simulink model "MIMO_model"  (R2018b)
settings: Solver=FixedStepAuto  StartTime=0.0  StopTime=Tmod  FixedStep=0.01  RelTol=1e-3
values from neighbouring files (symbols this model uses):
  denominator11 = FormDenominator(T1_11, T2_11, T3_11, flag11)    [Graph.m]    (also in KombRegNominalOU.m = FormDenominator(T1, T2, T3, flag); KombRobAdReg.m; KombRobReg.m; MIMONominalReg.m)
  denominator12 = FormDenominator(T1_12, T2_12, T3_12, flag12)    [Graph.m]    (also in KombRegNominalOU.m = FormDenominator(T1, T2, T3, flag); KombRobAdReg.m; KombRobReg.m; MIMONominalReg.m)
  denominator21 = FormDenominator(T1_21, T2_21, T3_21, flag21)    [Graph.m]    (also in KombRegNominalOU.m = FormDenominator(T1, T2, T3, flag); KombRobAdReg.m; KombRobReg.m; MIMONominalReg.m)
  denominator22 = FormDenominator(T1_22, T2_22, T3_22, flag22)    [Graph.m]    (also in KombRegNominalOU.m = FormDenominator(T1, T2, T3, flag); KombRobAdReg.m; KombRobReg.m; MIMONominalReg.m)
  ki11 = handles.savedValueWkiMS(1, 1)    [Graph.m]    (also in KombRegNominalOU.m = (ro_min *  (Wavt_Ki_Nom(1,1))) + ((1 - ro_min) * (Wvsp_Kp_No; KombRobAdReg.m = Wki_robast(1,1); KombRobReg.m = (ro_min_max *  (Wavt_Ki_Rob(1,1))) + ((1 - ro_min_max) * (Wv; MIMONominalReg.m = Wki_nominal(1,1))
  ki12 = handles.savedValueWkiMS(1, 2)    [Graph.m]    (also in KombRegNominalOU.m = (1 - ro_min) * (Wvsp_Ki_Nom(1,2)); KombRobAdReg.m = Wki_robast(1,2); KombRobReg.m = (1 - ro_min_max) * (Wvsp_Ki_Rob(1,2)); MIMONominalReg.m = Wki_nominal(1,2))
  ki21 = handles.savedValueWkiMS(2, 1)    [Graph.m]    (also in KombRegNominalOU.m = (1 - ro_min) * (Wvsp_Ki_Nom(2,1)); KombRobAdReg.m = Wki_robast(2,1); KombRobReg.m = (1 - ro_min_max) * (Wvsp_Ki_Rob(2,1)); MIMONominalReg.m = Wki_nominal(2,1))
  ki22 = handles.savedValueWkiMS(2, 2)    [Graph.m]    (also in KombRegNominalOU.m = ro_min * (Wavt_Ki_Nom(2,2)) + ((1 - ro_min) * (Wvsp_Ki_Nom(2; KombRobAdReg.m = Wki_robast(2,2); KombRobReg.m = ro_min_max * (Wavt_Ki_Rob(2,2)) + ((1 - ro_min_max) * (Wvsp_; MIMONominalReg.m = Wki_nominal(2,2))
  kp11 = handles.savedValueWkpMS(1, 1)    [Graph.m]    (also in KombRegNominalOU.m = (ro_min * (Wavt_Kp_Nom(1,1))) + ((1 - ro_min) * (Wvsp_Kp_Nom; KombRobAdReg.m = Wkp_robast(1,1); KombRobReg.m = (ro_min_max * (Wavt_Kp_Rob(1,1))) + ((1 - ro_min_max) * (Wvs; MIMONominalReg.m = Wkp_nominal(1,1))
  kp12 = handles.savedValueWkpMS(1, 2)    [Graph.m]    (also in KombRegNominalOU.m = (1 - ro_min) * (Wvsp_Kp_Nom(1,2)); KombRobAdReg.m = Wkp_robast(1,2); KombRobReg.m = (1 - ro_min_max) * (Wvsp_Kp_Rob(1,2)); MIMONominalReg.m = Wkp_nominal(1,2))
  kp21 = handles.savedValueWkpMS(2, 1)    [Graph.m]    (also in KombRegNominalOU.m = (1 - ro_min) * (Wvsp_Kp_Nom(2,1)); KombRobAdReg.m = Wkp_robast(2,1); KombRobReg.m = (1 - ro_min_max) * (Wvsp_Kp_Rob(2,1)); MIMONominalReg.m = Wkp_nominal(2,1))
  kp22 = handles.savedValueWkpMS(2, 2)    [Graph.m]    (also in KombRegNominalOU.m = ro_min * (Wavt_Kp_Nom(2,2)) + ((1 - ro_min) * (Wvsp_Kp_Nom(2; KombRobAdReg.m = Wkp_robast(2,2); KombRobReg.m = ro_min_max * (Wavt_Kp_Rob(2,2)) + ((1 - ro_min_max) * (Wvsp_; MIMONominalReg.m = Wkp_nominal(2,2))
  numerator11 = FormNumerator(k11, k11_2)    [Graph.m]    (also in KombRegNominalOU.m = FormNumerator(k, k2); KombRobAdReg.m; KombRobReg.m; MIMONominalReg.m)
  numerator12 = FormNumerator(k12, k12_2)    [Graph.m]    (also in KombRegNominalOU.m = FormNumerator(k, k2); KombRobAdReg.m; KombRobReg.m; MIMONominalReg.m)
  numerator21 = FormNumerator(k21, k21_2)    [Graph.m]    (also in KombRegNominalOU.m = FormNumerator(k, k2); KombRobAdReg.m; KombRobReg.m; MIMONominalReg.m)
  numerator22 = FormNumerator(k22, k22_2)    [Graph.m]    (also in KombRegNominalOU.m = FormNumerator(k, k2); KombRobAdReg.m; KombRobReg.m; MIMONominalReg.m)
  tau11 = tau11_grid(idx)    [KombRobAdReg.m]    (also in KombRobReg.m; MIMONominalReg.m)
  tau12 = tau12_grid(idx)    [KombRobAdReg.m]    (also in KombRobReg.m; MIMONominalReg.m)
  tau21 = tau21_grid(idx)    [KombRobAdReg.m]    (also in KombRobReg.m; MIMONominalReg.m)
  tau22 = tau22_grid(idx)    [KombRobAdReg.m]    (also in KombRobReg.m; MIMONominalReg.m)
  Tmod = 500    [Approximation.m]    (also in ApproximationUncertainty.m; Main.m = 100; MainMenu.m = numericValueTmod)
undefined symbols (not defined in the file or in its folder): disturbance1, disturbance2
settings Model: Creator=stepa  LastModifiedBy=stepa

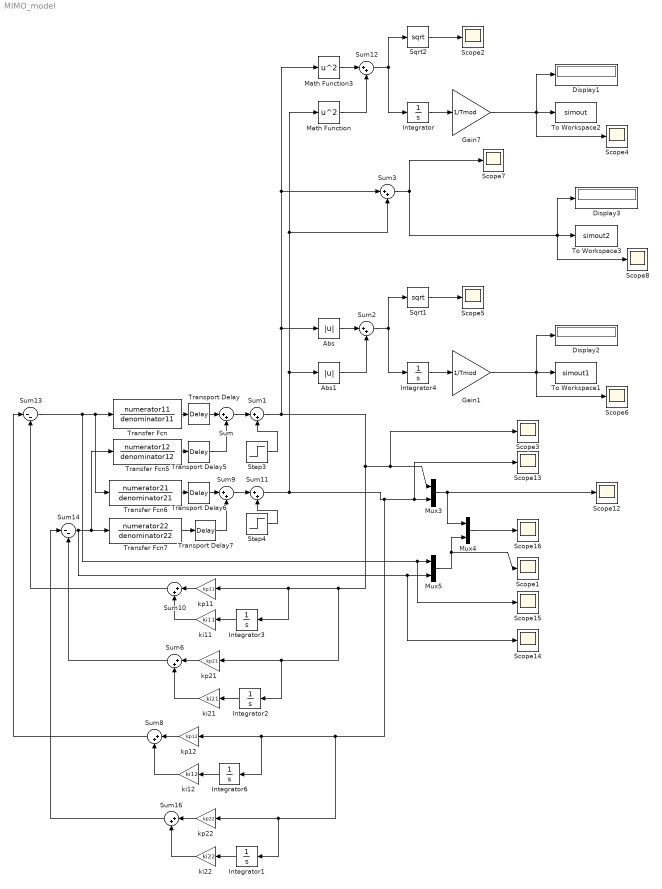
== system MIMO_model ==
  Abs : Abs
  Abs1 : Abs
  Display1 : Display
  Display2 : Display
  Display3 : Display
  Gain1 : Gain  Gain=1/Tmod
  Gain7 : Gain  Gain=1/Tmod
  Integrator{,1..4,6} (6 alike) : Integrator
  Math Function : Math  Operator=square  SaturateOnIntegerOverflow=on
  Math Function3 : Math  Operator=square  SaturateOnIntegerOverflow=on
  Mux3 : Mux  Inputs=2
  Mux4 : Mux  Inputs=2
  Mux5 : Mux  Inputs=2
  Scope{1..8,12..16} (13 alike) : Scope
  Sqrt1 : Sqrt  SaturateOnIntegerOverflow=on
  Sqrt2 : Sqrt  SaturateOnIntegerOverflow=on
  Step3 : Step  After=disturbance1  SampleTime=0
  Step4 : Step  After=disturbance2  SampleTime=0
  Sum{,1..3,6,8..12,16} (11 alike) : Sum  Inputs=|++
  Sum13 : Sum  Inputs=|--
  Sum14 : Sum  Inputs=|--
  To Workspace1 : ToWorkspace  VariableName=simout1  SampleTime=-1
      settings: MaxDataPoints=1
  To Workspace2 : ToWorkspace  VariableName=simout  SampleTime=-1
      settings: MaxDataPoints=1
  To Workspace3 : ToWorkspace  VariableName=simout2  SampleTime=-1
      settings: MaxDataPoints=50000
  Transfer Fcn : TransferFcn  Numerator=numerator11  Denominator=denominator11
  Transfer Fcn5 : TransferFcn  Numerator=numerator12  Denominator=denominator12
  Transfer Fcn6 : TransferFcn  Numerator=numerator21  Denominator=denominator21
  Transfer Fcn7 : TransferFcn  Numerator=numerator22  Denominator=denominator22
  Transport Delay : TransportDelay  DelayTime=tau11
  Transport Delay5 : TransportDelay  DelayTime=tau12
  Transport Delay6 : TransportDelay  DelayTime=tau21
  Transport Delay7 : TransportDelay  DelayTime=tau22
  ki11 : Gain  Gain=ki11
  ki12 : Gain  Gain=ki12
  ki21 : Gain  Gain=ki21
  ki22 : Gain  Gain=ki22
  kp11 : Gain  Gain=kp11
  "kp12 " : Gain  Gain=kp12
  kp21 : Gain  Gain=kp21
  kp22 : Gain  Gain=kp22
  wires:
  "kp12 "/1 -> Sum8/1
  Integrator/1 -> Gain7/1
  Sum8/1 -> Sum13/1
  ki12/1 -> Sum8/2
  kp11/1 -> Sum10/1
  Integrator6/1 -> ki12/1
  Integrator3/1 -> ki11/1
  Sqrt2/1 -> Scope2/1
  Transport Delay6/1 -> Sum9/1
  Mux5/1 -> Mux4/2, Scope1/1
  Integrator1/1 -> ki22/1
  Sum14/1 -> Transfer Fcn7/1, Transfer Fcn5/1, Scope14/1, Mux5/2
  ki21/1 -> Sum6/2
  Transport Delay/1 -> Sum/1
  Transport Delay7/1 -> Sum9/2
  Sum9/1 -> Sum11/1
  Step3/1 -> Sum1/2
  kp22/1 -> Sum16/1
  Transfer Fcn7/1 -> Transport Delay7/1
  Transfer Fcn6/1 -> Transport Delay6/1
  Sum16/1 -> Sum14/1
  Gain7/1 -> Scope4/1, To Workspace2/1, Display1/1
  Mux4/1 -> Scope16/1
  Transport Delay5/1 -> Sum/2
  kp21/1 -> Sum6/1
  Transfer Fcn/1 -> Transport Delay/1
  Transfer Fcn5/1 -> Transport Delay5/1
  Sum/1 -> Sum1/1
  Math Function3/1 -> Sum12/1
  Sum12/1 -> Integrator/1, Sqrt2/1
  Math Function/1 -> Sum12/2
  Integrator2/1 -> ki21/1
  ki22/1 -> Sum16/2
  ki11/1 -> Sum10/2
  Step4/1 -> Sum11/2
  Sum10/1 -> Sum13/2
  Sum13/1 -> Transfer Fcn6/1, Transfer Fcn/1, Scope15/1, Mux5/1
  Sum6/1 -> Sum14/2
  Sum2/1 -> Integrator4/1, Sqrt1/1
  Abs1/1 -> Sum2/2
  Gain1/1 -> Scope6/1, To Workspace1/1, Display2/1
  Sqrt1/1 -> Scope5/1
  Abs/1 -> Sum2/1
  Integrator4/1 -> Gain1/1
  Sum11/1 -> Abs1/1, Sum3/2, Math Function/1, "kp12 "/1, Integrator6/1, kp22/1, Integrator1/1, Scope13/1, Mux3/2
  Sum1/1 -> Abs/1, Math Function3/1, Sum3/1, Integrator3/1, kp11/1, Integrator2/1, kp21/1, Scope3/1, Mux3/1
  Sum3/1 -> Scope8/1, To Workspace3/1, Display3/1, Scope7/1
  Mux3/1 -> Mux4/1, Scope12/1
